simulink model "controller_traj_lin"  (R2025b)
settings: Solver=VariableStepAuto  StartTime=0.0  StopTime=10.0  RelTol=1e-3
settings Model: Creator=noyan  LastModifiedBy=noyan

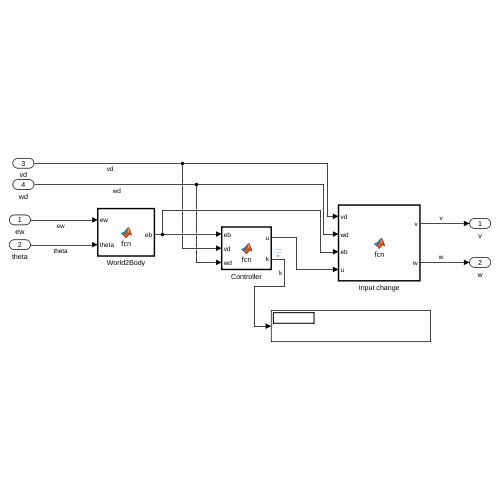
[thumbnail: Simulink's stored preview of the top-level diagram]
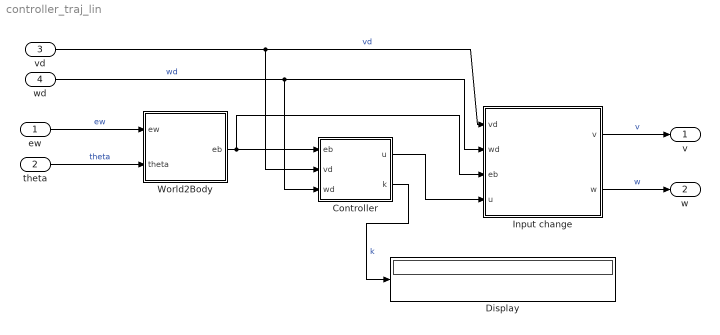
== system controller_traj_lin ==
  ew : Inport  PortDimensions=3
  theta : Inport  Port=2
  vd : Inport  Port=3
  wd : Inport  Port=4
  Controller : MATLAB Function  TreatAsAtomicUnit=on
  Display : Display
  Input change : MATLAB Function  TreatAsAtomicUnit=on
  World2Body : MATLAB Function  TreatAsAtomicUnit=on
  v : Outport
  w : Outport  Port=2
  wires:
  theta/1 -> World2Body/2(theta)  "theta"
  Controller/1(u) -> Input change/4(u)
  World2Body/1(eb) -> Controller/1(eb), Input change/3(eb)
  Input change/2(w) -> w/1  "w"
  ew/1 -> World2Body/1(ew)  "ew"
  Input change/1(v) -> v/1  "v"
  vd/1 -> Controller/2(vd), Input change/1(vd)  "vd"
  wd/1 -> Input change/2(wd), Controller/3(wd)  "wd"
  Controller/2(k) -> Display/1  "k"

== matlab function controller_traj_lin/World2Body ==
  data: ew input; eb output; theta input
function eb = fcn(ew, theta)
theta = wrapToPi(theta);
ew(3) = wrapToPi(ew(3));
Rbw = [cos(theta), -sin(theta); sin(theta), cos(theta)]'; % world to body
eb = [Rbw, [0; 0]; 0, 0, 1] * ew;
eb(3) = wrapToPi(eb(3));

== matlab function controller_traj_lin/Input change ==
  data: vd input; v output; wd input; eb input; u input; w output
function [v, w] = fcn(vd, wd, eb, u)
v = vd * cos(eb(3)) - u(1);
w = wd - u(2);
end

== matlab function controller_traj_lin/Controller ==
  data: eb input; u output; vd input; wd input; k output
function [u, k]= fcn(eb, vd, wd)
k = calculate_gains_traj_lin(vd, wd);

% u1 = -k(1) * eb(1);
% u2 = -k(2) * eb(2) - k(3) * eb(3);
% u = [u1, u2];

u = -k * eb;
end
